simulink library "LibFactorGraph"  (Simulink 8.3)
settings: Solver=ode45  StartTime=0.0  StopTime=10.0  RelTol=1e-3
undefined symbols (not defined in the file or in its folder): bV, epsVal, eu, fcn, fP_0, fV, Hin_0, L_0, Nit_0, P_0, xi
libraries: LibFactorGraph x357
(part 3 of 4)

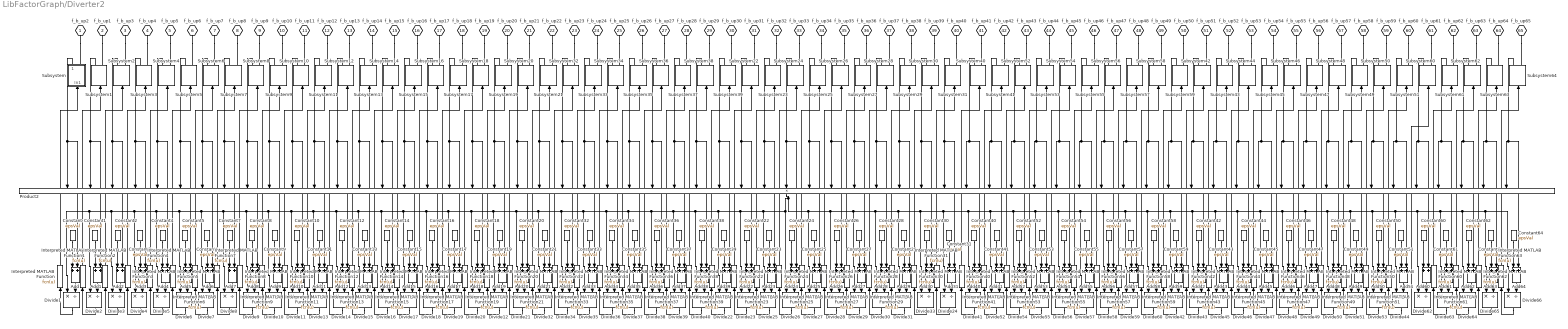
== system LibFactorGraph/Diverter2 ==
  Add{,1..64} (65 alike) : Sum
  Constant{,1..64} (65 alike) : Constant  Value=epsVal
  Divide{1..60,62..66} (65 alike) : Product  Inputs=*/
  Interpreted MATLAB Function{,1..63} (64 alike) : MATLABFcn  MATLABFcn=fcn(u)  Output1D=off
  Product2 : Product  Inputs=65  RndMeth=Zero
  Subsystem : Subsystem
  Subsystem{1..64} (64 alike) : LibFactorGraph/Diverter2/Subsystem
  f_b_up2 : PMIOPort  Port=1  Side=Left
  f_b_up1 : PMIOPort  Port=2  Side=Right
  f_b_up3 : PMIOPort  Port=3  Side=Left
  f_b_up4 : PMIOPort  Port=4  Side=Right
  f_b_up5 : PMIOPort  Port=5  Side=Left
  f_b_up6 : PMIOPort  Port=6  Side=Right
  f_b_up7 : PMIOPort  Port=7  Side=Left
  f_b_up8 : PMIOPort  Port=8  Side=Right
  f_b_up9 : PMIOPort  Port=9  Side=Left
  f_b_up10 : PMIOPort  Port=10  Side=Right
  f_b_up11 : PMIOPort  Port=11  Side=Left
  f_b_up12 : PMIOPort  Port=12  Side=Right
  f_b_up13 : PMIOPort  Port=13  Side=Left
  f_b_up14 : PMIOPort  Port=14  Side=Right
  f_b_up15 : PMIOPort  Port=15  Side=Left
  f_b_up16 : PMIOPort  Port=16  Side=Right
  f_b_up17 : PMIOPort  Port=17  Side=Left
  f_b_up18 : PMIOPort  Port=18  Side=Right
  f_b_up19 : PMIOPort  Port=19  Side=Left
  f_b_up20 : PMIOPort  Port=20  Side=Right
  f_b_up21 : PMIOPort  Port=21  Side=Left
  f_b_up22 : PMIOPort  Port=22  Side=Right
  f_b_up23 : PMIOPort  Port=23  Side=Left
  f_b_up24 : PMIOPort  Port=24  Side=Right
  f_b_up25 : PMIOPort  Port=25  Side=Left
  f_b_up26 : PMIOPort  Port=26  Side=Right
  f_b_up27 : PMIOPort  Port=27  Side=Left
  f_b_up28 : PMIOPort  Port=28  Side=Right
  f_b_up29 : PMIOPort  Port=29  Side=Left
  f_b_up30 : PMIOPort  Port=30  Side=Right
  f_b_up31 : PMIOPort  Port=31  Side=Left
  f_b_up32 : PMIOPort  Port=32  Side=Right
  f_b_up33 : PMIOPort  Port=33  Side=Left
  f_b_up34 : PMIOPort  Port=34  Side=Right
  f_b_up35 : PMIOPort  Port=35  Side=Left
  f_b_up36 : PMIOPort  Port=36  Side=Right
  f_b_up37 : PMIOPort  Port=37  Side=Left
  f_b_up38 : PMIOPort  Port=38  Side=Right
  f_b_up39 : PMIOPort  Port=39  Side=Left
  f_b_up40 : PMIOPort  Port=40  Side=Right
  f_b_up41 : PMIOPort  Port=41  Side=Left
  f_b_up42 : PMIOPort  Port=42  Side=Right
  f_b_up43 : PMIOPort  Port=43  Side=Left
  f_b_up44 : PMIOPort  Port=44  Side=Right
  f_b_up45 : PMIOPort  Port=45  Side=Left
  f_b_up46 : PMIOPort  Port=46  Side=Right
  f_b_up47 : PMIOPort  Port=47  Side=Left
  f_b_up48 : PMIOPort  Port=48  Side=Right
  f_b_up49 : PMIOPort  Port=49  Side=Left
  f_b_up50 : PMIOPort  Port=50  Side=Right
  f_b_up51 : PMIOPort  Port=51  Side=Left
  f_b_up52 : PMIOPort  Port=52  Side=Right
  f_b_up53 : PMIOPort  Port=53  Side=Left
  f_b_up54 : PMIOPort  Port=54  Side=Right
  f_b_up55 : PMIOPort  Port=55  Side=Left
  f_b_up56 : PMIOPort  Port=56  Side=Right
  f_b_up57 : PMIOPort  Port=57  Side=Left
  f_b_up58 : PMIOPort  Port=58  Side=Right
  f_b_up59 : PMIOPort  Port=59  Side=Left
  f_b_up60 : PMIOPort  Port=60  Side=Right
  f_b_up61 : PMIOPort  Port=61  Side=Left
  f_b_up62 : PMIOPort  Port=62  Side=Right
  f_b_up63 : PMIOPort  Port=63  Side=Left
  f_b_up64 : PMIOPort  Port=64  Side=Right
  f_b_up65 : PMIOPort  Port=65  Side=Left
  wires:
  Divide1/1 -> Interpreted MATLAB Function/1
  Subsystem/1(Out1) -> Product2/1, Add/2
  Interpreted MATLAB Function/1 -> Subsystem/1(In1)
  Add/1 -> Divide1/2
  Constant/1 -> Add/1
  Divide2/1 -> Interpreted MATLAB Function1/1
  Subsystem1/1 -> Product2/2, Add1/2
  Interpreted MATLAB Function1/1 -> Subsystem1/1
  Add1/1 -> Divide2/2
  Constant1/1 -> Add1/1
  Product2/1 -> Divide25/1, Divide23/1, Divide22/1, Divide40/1, Divide39/1, Divide38/1, Divide37/1, Divide36/1, Divide35/1, Divide34/1, Divide32/1, Divide21/1, Divide12/1, Divide20/1, Divide19/1, Divide18/1, Divide17/1, Divide16/1, Divide15/1, Divide14/1, Divide13/1, Divide11/1, Divide10/1, Divide9/1, Divide8/1, Divide7/1, Divide6/1, Divide5/1, Divide4/1, Divide3/1, Divide2/1, Divide1/1, Divide26/1, Divide27/1, Divide28/1, Divide29/1, Divide30/1, Divide31/1, Divide33/1, Divide24/1, Divide41/1, Divide52/1, Divide54/1, Divide55/1, Divide56/1, Divide58/1, Divide59/1, Divide60/1, Divide42/1, Divide43/1, Divide45/1, Divide46/1, Divide47/1, Divide48/1, Divide49/1, Divide50/1, Divide51/1, Divide53/1, Divide44/1, Divide62/1, Divide63/1, Divide64/1, Divide65/1, Divide66/1, Divide57/1
  Divide3/1 -> Interpreted MATLAB Function2/1
  Subsystem2/1 -> Product2/3, Add2/2
  Interpreted MATLAB Function2/1 -> Subsystem2/1
  Add2/1 -> Divide3/2
  Constant2/1 -> Add2/1
  Divide4/1 -> Interpreted MATLAB Function3/1
  Subsystem3/1 -> Product2/4, Add3/2
  Interpreted MATLAB Function3/1 -> Subsystem3/1
  Add3/1 -> Divide4/2
  Constant3/1 -> Add3/1
  Divide5/1 -> Interpreted MATLAB Function4/1
  Subsystem4/1 -> Product2/5, Add4/2
  Interpreted MATLAB Function4/1 -> Subsystem4/1
  Add4/1 -> Divide5/2
  Constant4/1 -> Add4/1
  Divide6/1 -> Interpreted MATLAB Function5/1
  Subsystem5/1 -> Product2/6, Add5/2
  Interpreted MATLAB Function5/1 -> Subsystem5/1
  Add5/1 -> Divide6/2
  Constant5/1 -> Add5/1
  Divide7/1 -> Interpreted MATLAB Function6/1
  Subsystem6/1 -> Product2/7, Add6/2
  Interpreted MATLAB Function6/1 -> Subsystem6/1
  Add6/1 -> Divide7/2
  Constant6/1 -> Add6/1
  Divide8/1 -> Interpreted MATLAB Function7/1
  Subsystem7/1 -> Product2/8, Add7/2
  Interpreted MATLAB Function7/1 -> Subsystem7/1
  Add7/1 -> Divide8/2
  Constant7/1 -> Add7/1
  Divide9/1 -> Interpreted MATLAB Function8/1
  Subsystem8/1 -> Product2/9, Add8/2
  Interpreted MATLAB Function8/1 -> Subsystem8/1
  Add8/1 -> Divide9/2
  Constant8/1 -> Add8/1
  Divide10/1 -> Interpreted MATLAB Function9/1
  Subsystem9/1 -> Product2/10, Add9/2
  Interpreted MATLAB Function9/1 -> Subsystem9/1
  Add9/1 -> Divide10/2
  Constant9/1 -> Add9/1
  Divide11/1 -> Interpreted MATLAB Function10/1
  Subsystem10/1 -> Product2/11, Add10/2
  Interpreted MATLAB Function10/1 -> Subsystem10/1
  Add10/1 -> Divide11/2
  Constant10/1 -> Add10/1
  Divide13/1 -> Interpreted MATLAB Function11/1
  Subsystem11/1 -> Product2/12, Add11/2
  Interpreted MATLAB Function11/1 -> Subsystem11/1
  Add11/1 -> Divide13/2
  Constant11/1 -> Add11/1
  Divide14/1 -> Interpreted MATLAB Function12/1
  Subsystem12/1 -> Product2/13, Add12/2
  Interpreted MATLAB Function12/1 -> Subsystem12/1
  Add12/1 -> Divide14/2
  Constant12/1 -> Add12/1
  Divide15/1 -> Interpreted MATLAB Function13/1
  Subsystem13/1 -> Product2/14, Add13/2
  Interpreted MATLAB Function13/1 -> Subsystem13/1
  Add13/1 -> Divide15/2
  Constant13/1 -> Add13/1
  Divide16/1 -> Interpreted MATLAB Function14/1
  Subsystem14/1 -> Product2/15, Add14/2
  Interpreted MATLAB Function14/1 -> Subsystem14/1
  Add14/1 -> Divide16/2
  Constant14/1 -> Add14/1
  Divide17/1 -> Interpreted MATLAB Function15/1
  Subsystem15/1 -> Product2/16, Add15/2
  Interpreted MATLAB Function15/1 -> Subsystem15/1
  Add15/1 -> Divide17/2
  Constant15/1 -> Add15/1
  Divide18/1 -> Interpreted MATLAB Function16/1
  Subsystem16/1 -> Product2/17, Add16/2
  Interpreted MATLAB Function16/1 -> Subsystem16/1
  Add16/1 -> Divide18/2
  Constant16/1 -> Add16/1
  Divide19/1 -> Interpreted MATLAB Function17/1
  Subsystem17/1 -> Product2/18, Add17/2
  Interpreted MATLAB Function17/1 -> Subsystem17/1
  Add17/1 -> Divide19/2
  Constant17/1 -> Add17/1
  Divide20/1 -> Interpreted MATLAB Function18/1
  Subsystem18/1 -> Product2/19, Add18/2
  Interpreted MATLAB Function18/1 -> Subsystem18/1
  Add18/1 -> Divide20/2
  Constant18/1 -> Add18/1
  Divide12/1 -> Interpreted MATLAB Function19/1
  Subsystem19/1 -> Product2/20, Add19/2
  Interpreted MATLAB Function19/1 -> Subsystem19/1
  Add19/1 -> Divide12/2
  Constant19/1 -> Add19/1
  Divide21/1 -> Interpreted MATLAB Function20/1
  Subsystem20/1 -> Product2/21, Add20/2
  Interpreted MATLAB Function20/1 -> Subsystem20/1
  Add20/1 -> Divide21/2
  Constant20/1 -> Add20/1
  Divide32/1 -> Interpreted MATLAB Function21/1
  Subsystem21/1 -> Product2/22, Add21/2
  Interpreted MATLAB Function21/1 -> Subsystem21/1
  Add21/1 -> Divide32/2
  Constant21/1 -> Add21/1
  Divide34/1 -> Interpreted MATLAB Function32/1
  Subsystem32/1 -> Product2/23, Add32/2
  Interpreted MATLAB Function32/1 -> Subsystem32/1
  Add32/1 -> Divide34/2
  Constant32/1 -> Add32/1
  Divide35/1 -> Interpreted MATLAB Function33/1
  Subsystem33/1 -> Product2/24, Add33/2
  Interpreted MATLAB Function33/1 -> Subsystem33/1
  Add33/1 -> Divide35/2
  Constant33/1 -> Add33/1
  Divide36/1 -> Interpreted MATLAB Function34/1
  Subsystem34/1 -> Product2/25, Add34/2
  Interpreted MATLAB Function34/1 -> Subsystem34/1
  Add34/1 -> Divide36/2
  Constant34/1 -> Add34/1
  Divide37/1 -> Interpreted MATLAB Function35/1
  Subsystem35/1 -> Product2/26, Add35/2
  Interpreted MATLAB Function35/1 -> Subsystem35/1
  Add35/1 -> Divide37/2
  Constant35/1 -> Add35/1
  Divide38/1 -> Interpreted MATLAB Function36/1
  Subsystem36/1 -> Product2/27, Add36/2
  Interpreted MATLAB Function36/1 -> Subsystem36/1
  Add36/1 -> Divide38/2
  Constant36/1 -> Add36/1
  Divide39/1 -> Interpreted MATLAB Function37/1
  Subsystem37/1 -> Product2/28, Add37/2
  Interpreted MATLAB Function37/1 -> Subsystem37/1
  Add37/1 -> Divide39/2
  Constant37/1 -> Add37/1
  Divide40/1 -> Interpreted MATLAB Function38/1
  Subsystem38/1 -> Product2/29, Add38/2
  Interpreted MATLAB Function38/1 -> Subsystem38/1
  Add38/1 -> Divide40/2
  Constant38/1 -> Add38/1
  Divide22/1 -> Interpreted MATLAB Function39/1
  Subsystem39/1 -> Product2/30, Add39/2
  Interpreted MATLAB Function39/1 -> Subsystem39/1
  Add39/1 -> Divide22/2
  Constant39/1 -> Add39/1
  Divide23/1 -> Interpreted MATLAB Function22/1
  Subsystem22/1 -> Product2/31, Add22/2
  Interpreted MATLAB Function22/1 -> Subsystem22/1
  Add22/1 -> Divide23/2
  Constant22/1 -> Add22/1
  Divide25/1 -> Interpreted MATLAB Function23/1
  Subsystem23/1 -> Product2/32, Add23/2
  Interpreted MATLAB Function23/1 -> Subsystem23/1
  Add23/1 -> Divide25/2
  Constant23/1 -> Add23/1
  Divide26/1 -> Interpreted MATLAB Function24/1
  Subsystem24/1 -> Product2/33, Add24/2
  Interpreted MATLAB Function24/1 -> Subsystem24/1
  Add24/1 -> Divide26/2
  Constant24/1 -> Add24/1
  Divide27/1 -> Interpreted MATLAB Function25/1
  Subsystem25/1 -> Product2/34, Add25/2
  Interpreted MATLAB Function25/1 -> Subsystem25/1
  Add25/1 -> Divide27/2
  Constant25/1 -> Add25/1
  Divide28/1 -> Interpreted MATLAB Function26/1
  Subsystem26/1 -> Product2/35, Add26/2
  Interpreted MATLAB Function26/1 -> Subsystem26/1
  Add26/1 -> Divide28/2
  Constant26/1 -> Add26/1
  Divide29/1 -> Interpreted MATLAB Function27/1
  Subsystem27/1 -> Product2/36, Add27/2
  Interpreted MATLAB Function27/1 -> Subsystem27/1
  Add27/1 -> Divide29/2
  Constant27/1 -> Add27/1
  Divide30/1 -> Interpreted MATLAB Function28/1
  Subsystem28/1 -> Product2/37, Add28/2
  Interpreted MATLAB Function28/1 -> Subsystem28/1
  Add28/1 -> Divide30/2
  Constant28/1 -> Add28/1
  Divide31/1 -> Interpreted MATLAB Function29/1
  Subsystem29/1 -> Product2/38, Add29/2
  Interpreted MATLAB Function29/1 -> Subsystem29/1
  Add29/1 -> Divide31/2
  Constant29/1 -> Add29/1
  Divide33/1 -> Interpreted MATLAB Function30/1
  Subsystem30/1 -> Product2/39, Add30/2
  Interpreted MATLAB Function30/1 -> Subsystem30/1
  Add30/1 -> Divide33/2
  Constant30/1 -> Add30/1
  Divide24/1 -> Interpreted MATLAB Function31/1
  Subsystem31/1 -> Product2/40, Add31/2
  Interpreted MATLAB Function31/1 -> Subsystem31/1
  Add31/1 -> Divide24/2
  Constant31/1 -> Add31/1
  Divide41/1 -> Interpreted MATLAB Function40/1
  Subsystem40/1 -> Product2/41, Add40/2
  Interpreted MATLAB Function40/1 -> Subsystem40/1
  Add40/1 -> Divide41/2
  Constant40/1 -> Add40/1
  Divide52/1 -> Interpreted MATLAB Function41/1
  Subsystem41/1 -> Product2/42, Add41/2
  Interpreted MATLAB Function41/1 -> Subsystem41/1
  Add41/1 -> Divide52/2
  Constant41/1 -> Add41/1
  Divide54/1 -> Interpreted MATLAB Function52/1
  Subsystem52/1 -> Product2/43, Add52/2
  Interpreted MATLAB Function52/1 -> Subsystem52/1
  Add52/1 -> Divide54/2
  Constant52/1 -> Add52/1
  Divide55/1 -> Interpreted MATLAB Function53/1
  Subsystem53/1 -> Product2/44, Add53/2
  Interpreted MATLAB Function53/1 -> Subsystem53/1
  Add53/1 -> Divide55/2
  Constant53/1 -> Add53/1
  Divide56/1 -> Interpreted MATLAB Function54/1
  Subsystem54/1 -> Product2/45, Add54/2
  Interpreted MATLAB Function54/1 -> Subsystem54/1
  Add54/1 -> Divide56/2
  Constant54/1 -> Add54/1
  Divide57/1 -> Interpreted MATLAB Function55/1
  Subsystem55/1 -> Product2/46, Add55/2
  Interpreted MATLAB Function55/1 -> Subsystem55/1
  Add55/1 -> Divide57/2
  Constant55/1 -> Add55/1
  Divide58/1 -> Interpreted MATLAB Function56/1
  Subsystem56/1 -> Product2/47, Add56/2
  Interpreted MATLAB Function56/1 -> Subsystem56/1
  Add56/1 -> Divide58/2
  Constant56/1 -> Add56/1
  Divide59/1 -> Interpreted MATLAB Function57/1
  Subsystem57/1 -> Product2/48, Add57/2
  Interpreted MATLAB Function57/1 -> Subsystem57/1
  Add57/1 -> Divide59/2
  Constant57/1 -> Add57/1
  Divide60/1 -> Interpreted MATLAB Function58/1
  Subsystem58/1 -> Product2/49, Add58/2
  Interpreted MATLAB Function58/1 -> Subsystem58/1
  Add58/1 -> Divide60/2
  Constant58/1 -> Add58/1
  Divide42/1 -> Interpreted MATLAB Function59/1
  Subsystem59/1 -> Product2/50, Add59/2
  Interpreted MATLAB Function59/1 -> Subsystem59/1
  Add59/1 -> Divide42/2
  Constant59/1 -> Add59/1
  Divide43/1 -> Interpreted MATLAB Function42/1
  Subsystem42/1 -> Product2/51, Add42/2
  Interpreted MATLAB Function42/1 -> Subsystem42/1
  Add42/1 -> Divide43/2
  Constant42/1 -> Add42/1
  Divide45/1 -> Interpreted MATLAB Function43/1
  Subsystem43/1 -> Product2/52, Add43/2
  Interpreted MATLAB Function43/1 -> Subsystem43/1
  Add43/1 -> Divide45/2
  Constant43/1 -> Add43/1
  Divide46/1 -> Interpreted MATLAB Function44/1
  Subsystem44/1 -> Product2/53, Add44/2
  Interpreted MATLAB Function44/1 -> Subsystem44/1
  Add44/1 -> Divide46/2
  Constant44/1 -> Add44/1
  Divide47/1 -> Interpreted MATLAB Function45/1
  Subsystem45/1 -> Product2/54, Add45/2
  Interpreted MATLAB Function45/1 -> Subsystem45/1
  Add45/1 -> Divide47/2
  Constant45/1 -> Add45/1
  Divide48/1 -> Interpreted MATLAB Function46/1
  Subsystem46/1 -> Product2/55, Add46/2
  Interpreted MATLAB Function46/1 -> Subsystem46/1
  Add46/1 -> Divide48/2
  Constant46/1 -> Add46/1
  Divide49/1 -> Interpreted MATLAB Function47/1
  Subsystem47/1 -> Product2/56, Add47/2
  Interpreted MATLAB Function47/1 -> Subsystem47/1
  Add47/1 -> Divide49/2
  Constant47/1 -> Add47/1
  Divide50/1 -> Interpreted MATLAB Function48/1
  Subsystem48/1 -> Product2/57, Add48/2
  Interpreted MATLAB Function48/1 -> Subsystem48/1
  Add48/1 -> Divide50/2
  Constant48/1 -> Add48/1
  Divide51/1 -> Interpreted MATLAB Function49/1
  Subsystem49/1 -> Product2/58, Add49/2
  Interpreted MATLAB Function49/1 -> Subsystem49/1
  Add49/1 -> Divide51/2
  Constant49/1 -> Add49/1
  Divide53/1 -> Interpreted MATLAB Function50/1
  Subsystem50/1 -> Product2/59, Add50/2
  Interpreted MATLAB Function50/1 -> Subsystem50/1
  Add50/1 -> Divide53/2
  Constant50/1 -> Add50/1
  Divide44/1 -> Interpreted MATLAB Function51/1
  Subsystem51/1 -> Product2/60, Add51/2
  Interpreted MATLAB Function51/1 -> Subsystem51/1
  Add51/1 -> Divide44/2
  Constant51/1 -> Add51/1
  Subsystem60/1 -> Product2/61, Add60/2
  Divide62/1 -> Subsystem60/1
  Add60/1 -> Divide62/2
  Constant60/1 -> Add60/1
  Divide63/1 -> Interpreted MATLAB Function60/1
  Subsystem61/1 -> Product2/62, Add61/2
  Interpreted MATLAB Function60/1 -> Subsystem61/1
  Add61/1 -> Divide63/2
  Constant61/1 -> Add61/1
  Divide64/1 -> Interpreted MATLAB Function61/1
  Subsystem62/1 -> Product2/63, Add62/2
  Interpreted MATLAB Function61/1 -> Subsystem62/1
  Add62/1 -> Divide64/2
  Constant62/1 -> Add62/1
  Divide65/1 -> Interpreted MATLAB Function62/1
  Subsystem63/1 -> Product2/64, Add63/2
  Interpreted MATLAB Function62/1 -> Subsystem63/1
  Add63/1 -> Divide65/2
  Constant63/1 -> Add63/1
  Divide66/1 -> Interpreted MATLAB Function63/1
  Subsystem64/1 -> Product2/65, Add64/2
  Interpreted MATLAB Function63/1 -> Subsystem64/1
  Add64/1 -> Divide66/2
  Constant64/1 -> Add64/1
  connections:
  f_b_up2/RConn1 -- Subsystem/RConn1
  f_b_up1/RConn1 -- Subsystem1/RConn1
  f_b_up3/RConn1 -- Subsystem2/RConn1
  f_b_up4/RConn1 -- Subsystem3/RConn1
  f_b_up5/RConn1 -- Subsystem4/RConn1
  f_b_up7/RConn1 -- Subsystem6/RConn1
  f_b_up6/RConn1 -- Subsystem5/RConn1
  f_b_up10/RConn1 -- Subsystem9/RConn1
  f_b_up8/RConn1 -- Subsystem7/RConn1
  f_b_up9/RConn1 -- Subsystem8/RConn1
  f_b_up16/RConn1 -- Subsystem15/RConn1
  f_b_up14/RConn1 -- Subsystem13/RConn1
  f_b_up12/RConn1 -- Subsystem11/RConn1
  f_b_up15/RConn1 -- Subsystem14/RConn1
  f_b_up19/RConn1 -- Subsystem18/RConn1
  f_b_up18/RConn1 -- Subsystem17/RConn1
  f_b_up11/RConn1 -- Subsystem10/RConn1
  f_b_up17/RConn1 -- Subsystem16/RConn1
  f_b_up20/RConn1 -- Subsystem19/RConn1
  f_b_up13/RConn1 -- Subsystem12/RConn1
  f_b_up36/RConn1 -- Subsystem27/RConn1
  f_b_up38/RConn1 -- Subsystem29/RConn1
  f_b_up26/RConn1 -- Subsystem35/RConn1
  f_b_up39/RConn1 -- Subsystem30/RConn1
  f_b_up23/RConn1 -- Subsystem32/RConn1
  f_b_up34/RConn1 -- Subsystem25/RConn1
  f_b_up27/RConn1 -- Subsystem36/RConn1
  f_b_up25/RConn1 -- Subsystem34/RConn1
  f_b_up31/RConn1 -- Subsystem22/RConn1
  f_b_up24/RConn1 -- Subsystem33/RConn1
  f_b_up22/RConn1 -- Subsystem21/RConn1
  f_b_up28/RConn1 -- Subsystem37/RConn1
  f_b_up37/RConn1 -- Subsystem28/RConn1
  f_b_up33/RConn1 -- Subsystem24/RConn1
  f_b_up30/RConn1 -- Subsystem39/RConn1
  f_b_up35/RConn1 -- Subsystem26/RConn1
  f_b_up21/RConn1 -- Subsystem20/RConn1
  f_b_up32/RConn1 -- Subsystem23/RConn1
  f_b_up40/RConn1 -- Subsystem31/RConn1
  f_b_up29/RConn1 -- Subsystem38/RConn1
  f_b_up56/RConn1 -- Subsystem47/RConn1
  f_b_up58/RConn1 -- Subsystem49/RConn1
  f_b_up46/RConn1 -- Subsystem55/RConn1
  f_b_up59/RConn1 -- Subsystem50/RConn1
  f_b_up43/RConn1 -- Subsystem52/RConn1
  f_b_up54/RConn1 -- Subsystem45/RConn1
  f_b_up47/RConn1 -- Subsystem56/RConn1
  f_b_up45/RConn1 -- Subsystem54/RConn1
  f_b_up51/RConn1 -- Subsystem42/RConn1
  f_b_up44/RConn1 -- Subsystem53/RConn1
  f_b_up42/RConn1 -- Subsystem41/RConn1
  f_b_up48/RConn1 -- Subsystem57/RConn1
  f_b_up57/RConn1 -- Subsystem48/RConn1
  f_b_up53/RConn1 -- Subsystem44/RConn1
  f_b_up50/RConn1 -- Subsystem59/RConn1
  f_b_up55/RConn1 -- Subsystem46/RConn1
  f_b_up41/RConn1 -- Subsystem40/RConn1
  f_b_up52/RConn1 -- Subsystem43/RConn1
  f_b_up60/RConn1 -- Subsystem51/RConn1
  f_b_up49/RConn1 -- Subsystem58/RConn1
  f_b_up63/RConn1 -- Subsystem62/RConn1
  f_b_up64/RConn1 -- Subsystem63/RConn1
  f_b_up62/RConn1 -- Subsystem61/RConn1
  f_b_up65/RConn1 -- Subsystem64/RConn1
  f_b_up61/RConn1 -- Subsystem60/RConn1

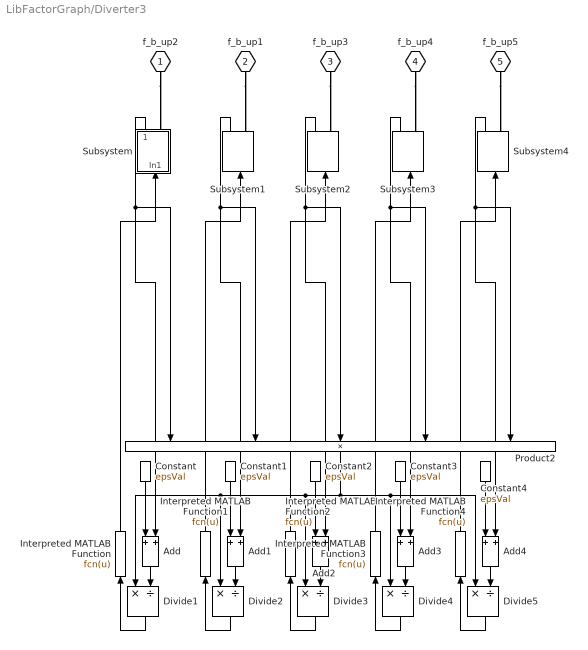
== system LibFactorGraph/Diverter3 ==
  Add{,1..4} (5 alike) : Sum
  Constant{,1..4} (5 alike) : Constant  Value=epsVal
  Divide{1..5} (5 alike) : Product  Inputs=*/
  Interpreted MATLAB Function{,1..4} (5 alike) : MATLABFcn  MATLABFcn=fcn(u)  Output1D=off
  Product2 : Product  Inputs=5  RndMeth=Zero
  Subsystem : Subsystem
  Subsystem{1..4} (4 alike) : LibFactorGraph/Diverter3/Subsystem
  f_b_up2 : PMIOPort  Port=1  Side=Left
  f_b_up1 : PMIOPort  Port=2  Side=Right
  f_b_up3 : PMIOPort  Port=3  Side=Left
  f_b_up4 : PMIOPort  Port=4  Side=Right
  f_b_up5 : PMIOPort  Port=5  Side=Left
  wires:
  Constant/1 -> Add/1
  Add/1 -> Divide1/2
  Interpreted MATLAB Function/1 -> Subsystem/1(In1)
  Subsystem/1(Out1) -> Add/2, Product2/1
  Divide1/1 -> Interpreted MATLAB Function/1
  Constant1/1 -> Add1/1
  Add1/1 -> Divide2/2
  Interpreted MATLAB Function1/1 -> Subsystem1/1
  Subsystem1/1 -> Product2/2, Add1/2
  Divide2/1 -> Interpreted MATLAB Function1/1
  Constant2/1 -> Add2/1
  Add2/1 -> Divide3/2
  Interpreted MATLAB Function2/1 -> Subsystem2/1
  Subsystem2/1 -> Product2/3, Add2/2
  Divide3/1 -> Interpreted MATLAB Function2/1
  Constant3/1 -> Add3/1
  Add3/1 -> Divide4/2
  Interpreted MATLAB Function3/1 -> Subsystem3/1
  Subsystem3/1 -> Product2/4, Add3/2
  Divide4/1 -> Interpreted MATLAB Function3/1
  Product2/1 -> Divide2/1, Divide1/1, Divide3/1, Divide5/1, Divide4/1
  Constant4/1 -> Add4/1
  Add4/1 -> Divide5/2
  Interpreted MATLAB Function4/1 -> Subsystem4/1
  Subsystem4/1 -> Product2/5, Add4/2
  Divide5/1 -> Interpreted MATLAB Function4/1
  connections:
  f_b_up2/RConn1 -- Subsystem/RConn1
  f_b_up1/RConn1 -- Subsystem1/RConn1
  f_b_up3/RConn1 -- Subsystem2/RConn1
  f_b_up4/RConn1 -- Subsystem3/RConn1
  f_b_up5/RConn1 -- Subsystem4/RConn1

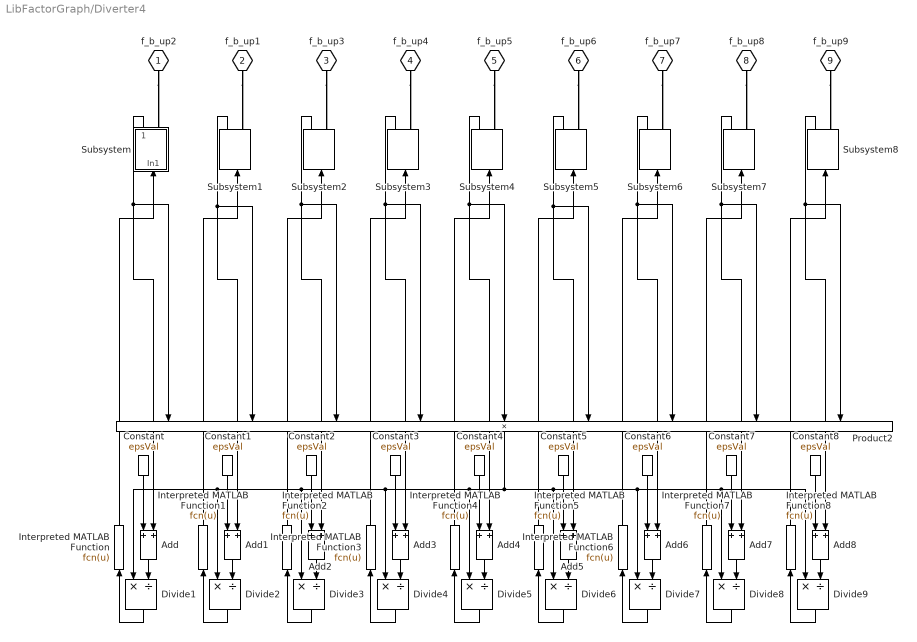
== system LibFactorGraph/Diverter4 ==
  Add{,1..8} (9 alike) : Sum
  Constant{,1..8} (9 alike) : Constant  Value=epsVal
  Divide{1..9} (9 alike) : Product  Inputs=*/
  Interpreted MATLAB Function{,1..8} (9 alike) : MATLABFcn  MATLABFcn=fcn(u)  Output1D=off
  Product2 : Product  Inputs=9  RndMeth=Zero
  Subsystem : Subsystem
  Subsystem{1..3,5..8} (7 alike) : LibFactorGraph/Diverter3/Subsystem
  Subsystem4 : LibFactorGraph/Diverter4/Subsystem
  f_b_up2 : PMIOPort  Port=1  Side=Left
  f_b_up1 : PMIOPort  Port=2  Side=Right
  f_b_up3 : PMIOPort  Port=3  Side=Left
  f_b_up4 : PMIOPort  Port=4  Side=Right
  f_b_up5 : PMIOPort  Port=5  Side=Left
  f_b_up6 : PMIOPort  Port=6  Side=Right
  f_b_up7 : PMIOPort  Port=7  Side=Left
  f_b_up8 : PMIOPort  Port=8  Side=Right
  f_b_up9 : PMIOPort  Port=9  Side=Left
  wires:
  Divide4/1 -> Interpreted MATLAB Function3/1
  Subsystem3/1 -> Add3/2, Product2/4
  Interpreted MATLAB Function3/1 -> Subsystem3/1
  Add3/1 -> Divide4/2
  Constant3/1 -> Add3/1
  Divide3/1 -> Interpreted MATLAB Function2/1
  Subsystem2/1 -> Add2/2, Product2/3
  Interpreted MATLAB Function2/1 -> Subsystem2/1
  Add2/1 -> Divide3/2
  Constant2/1 -> Add2/1
  Divide2/1 -> Interpreted MATLAB Function1/1
  Subsystem1/1 -> Product2/2, Add1/2
  Interpreted MATLAB Function1/1 -> Subsystem1/1
  Add1/1 -> Divide2/2
  Constant1/1 -> Add1/1
  Divide1/1 -> Interpreted MATLAB Function/1
  Subsystem/1(Out1) -> Product2/1, Add/2
  Interpreted MATLAB Function/1 -> Subsystem/1(In1)
  Add/1 -> Divide1/2
  Constant/1 -> Add/1
  Divide8/1 -> Interpreted MATLAB Function7/1
  Subsystem7/1 -> Product2/8, Add7/2
  Interpreted MATLAB Function7/1 -> Subsystem7/1
  Add7/1 -> Divide8/2
  Constant7/1 -> Add7/1
  Divide7/1 -> Interpreted MATLAB Function6/1
  Subsystem6/1 -> Product2/7, Add6/2
  Interpreted MATLAB Function6/1 -> Subsystem6/1
  Add6/1 -> Divide7/2
  Constant6/1 -> Add6/1
  Divide6/1 -> Interpreted MATLAB Function5/1
  Subsystem5/1 -> Product2/6, Add5/2
  Interpreted MATLAB Function5/1 -> Subsystem5/1
  Add5/1 -> Divide6/2
  Constant5/1 -> Add5/1
  Divide5/1 -> Interpreted MATLAB Function4/1
  Subsystem4/1 -> Product2/5, Add4/2
  Interpreted MATLAB Function4/1 -> Subsystem4/1
  Add4/1 -> Divide5/2
  Constant4/1 -> Add4/1
  Divide9/1 -> Interpreted MATLAB Function8/1
  Subsystem8/1 -> Product2/9, Add8/2
  Interpreted MATLAB Function8/1 -> Subsystem8/1
  Add8/1 -> Divide9/2
  Constant8/1 -> Add8/1
  Product2/1 -> Divide5/1, Divide1/1, Divide2/1, Divide3/1, Divide4/1, Divide9/1, Divide8/1, Divide7/1, Divide6/1
  connections:
  f_b_up4/RConn1 -- Subsystem3/RConn1
  f_b_up3/RConn1 -- Subsystem2/RConn1
  f_b_up1/RConn1 -- Subsystem1/RConn1
  f_b_up2/RConn1 -- Subsystem/RConn1
  f_b_up5/RConn1 -- Subsystem4/RConn1
  f_b_up6/RConn1 -- Subsystem5/RConn1
  f_b_up8/RConn1 -- Subsystem7/RConn1
  f_b_up7/RConn1 -- Subsystem6/RConn1
  f_b_up9/RConn1 -- Subsystem8/RConn1

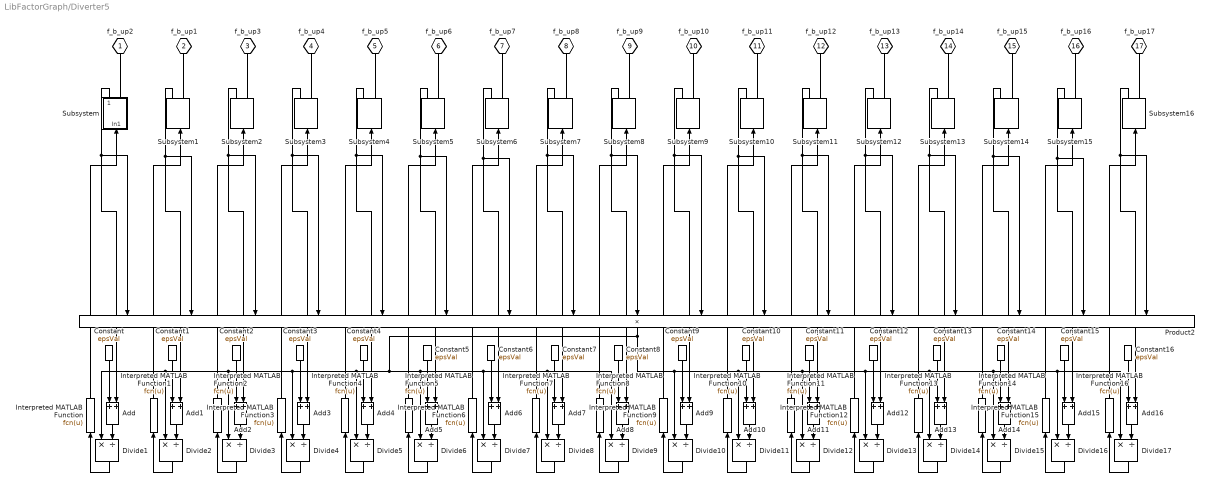
== system LibFactorGraph/Diverter5 ==
  Add{,1..16} (17 alike) : Sum
  Constant{,1..16} (17 alike) : Constant  Value=epsVal
  Divide{1..17} (17 alike) : Product  Inputs=*/
  Interpreted MATLAB Function{,1..16} (17 alike) : MATLABFcn  MATLABFcn=fcn(u)  Output1D=off
  Product2 : Product  Inputs=17  RndMeth=Zero
  Subsystem : Subsystem
  Subsystem{1..3,5..8,10..12,14..16} (13 alike) : LibFactorGraph/Diverter3/Subsystem
  Subsystem13 : LibFactorGraph/Diverter4/Subsystem
  Subsystem4 : LibFactorGraph/Diverter4/Subsystem
  Subsystem9 : LibFactorGraph/Diverter5/Subsystem
  f_b_up2 : PMIOPort  Port=1  Side=Left
  f_b_up1 : PMIOPort  Port=2  Side=Right
  f_b_up3 : PMIOPort  Port=3  Side=Left
  f_b_up4 : PMIOPort  Port=4  Side=Right
  f_b_up5 : PMIOPort  Port=5  Side=Left
  f_b_up6 : PMIOPort  Port=6  Side=Right
  f_b_up7 : PMIOPort  Port=7  Side=Left
  f_b_up8 : PMIOPort  Port=8  Side=Right
  f_b_up9 : PMIOPort  Port=9  Side=Left
  f_b_up10 : PMIOPort  Port=10  Side=Right
  f_b_up11 : PMIOPort  Port=11  Side=Left
  f_b_up12 : PMIOPort  Port=12  Side=Right
  f_b_up13 : PMIOPort  Port=13  Side=Left
  f_b_up14 : PMIOPort  Port=14  Side=Right
  f_b_up15 : PMIOPort  Port=15  Side=Left
  f_b_up16 : PMIOPort  Port=16  Side=Right
  f_b_up17 : PMIOPort  Port=17  Side=Left
  wires:
  Divide4/1 -> Interpreted MATLAB Function3/1
  Subsystem3/1 -> Add3/2, Product2/4
  Interpreted MATLAB Function3/1 -> Subsystem3/1
  Add3/1 -> Divide4/2
  Constant3/1 -> Add3/1
  Divide3/1 -> Interpreted MATLAB Function2/1
  Subsystem2/1 -> Add2/2, Product2/3
  Interpreted MATLAB Function2/1 -> Subsystem2/1
  Add2/1 -> Divide3/2
  Constant2/1 -> Add2/1
  Divide2/1 -> Interpreted MATLAB Function1/1
  Subsystem1/1 -> Product2/2, Add1/2
  Interpreted MATLAB Function1/1 -> Subsystem1/1
  Add1/1 -> Divide2/2
  Constant1/1 -> Add1/1
  Divide1/1 -> Interpreted MATLAB Function/1
  Subsystem/1(Out1) -> Product2/1, Add/2
  Interpreted MATLAB Function/1 -> Subsystem/1(In1)
  Add/1 -> Divide1/2
  Constant/1 -> Add/1
  Divide8/1 -> Interpreted MATLAB Function7/1
  Subsystem7/1 -> Product2/8, Add7/2
  Interpreted MATLAB Function7/1 -> Subsystem7/1
  Add7/1 -> Divide8/2
  Constant7/1 -> Add7/1
  Divide7/1 -> Interpreted MATLAB Function6/1
  Subsystem6/1 -> Product2/7, Add6/2
  Interpreted MATLAB Function6/1 -> Subsystem6/1
  Add6/1 -> Divide7/2
  Constant6/1 -> Add6/1
  Divide6/1 -> Interpreted MATLAB Function5/1
  Subsystem5/1 -> Product2/6, Add5/2
  Interpreted MATLAB Function5/1 -> Subsystem5/1
  Add5/1 -> Divide6/2
  Constant5/1 -> Add5/1
  Divide5/1 -> Interpreted MATLAB Function4/1
  Subsystem4/1 -> Product2/5, Add4/2
  Interpreted MATLAB Function4/1 -> Subsystem4/1
  Add4/1 -> Divide5/2
  Constant4/1 -> Add4/1
  Divide9/1 -> Interpreted MATLAB Function8/1
  Subsystem8/1 -> Product2/9, Add8/2
  Interpreted MATLAB Function8/1 -> Subsystem8/1
  Add8/1 -> Divide9/2
  Constant8/1 -> Add8/1
  Divide13/1 -> Interpreted MATLAB Function12/1
  Subsystem12/1 -> Product2/13, Add12/2
  Interpreted MATLAB Function12/1 -> Subsystem12/1
  Add12/1 -> Divide13/2
  Constant12/1 -> Add12/1
  Divide12/1 -> Interpreted MATLAB Function11/1
  Subsystem11/1 -> Product2/12, Add11/2
  Interpreted MATLAB Function11/1 -> Subsystem11/1
  Add11/1 -> Divide12/2
  Constant11/1 -> Add11/1
  Divide11/1 -> Interpreted MATLAB Function10/1
  Subsystem10/1 -> Product2/11, Add10/2
  Interpreted MATLAB Function10/1 -> Subsystem10/1
  Add10/1 -> Divide11/2
  Constant10/1 -> Add10/1
  Divide10/1 -> Interpreted MATLAB Function9/1
  Subsystem9/1 -> Product2/10, Add9/2
  Interpreted MATLAB Function9/1 -> Subsystem9/1
  Add9/1 -> Divide10/2
  Constant9/1 -> Add9/1
  Divide17/1 -> Interpreted MATLAB Function16/1
  Subsystem16/1 -> Product2/17, Add16/2
  Interpreted MATLAB Function16/1 -> Subsystem16/1
  Add16/1 -> Divide17/2
  Constant16/1 -> Add16/1
  Divide16/1 -> Interpreted MATLAB Function15/1
  Subsystem15/1 -> Product2/16, Add15/2
  Interpreted MATLAB Function15/1 -> Subsystem15/1
  Add15/1 -> Divide16/2
  Constant15/1 -> Add15/1
  Divide15/1 -> Interpreted MATLAB Function14/1
  Subsystem14/1 -> Product2/15, Add14/2
  Interpreted MATLAB Function14/1 -> Subsystem14/1
  Add14/1 -> Divide15/2
  Constant14/1 -> Add14/1
  Divide14/1 -> Interpreted MATLAB Function13/1
  Subsystem13/1 -> Product2/14, Add13/2
  Interpreted MATLAB Function13/1 -> Subsystem13/1
  Add13/1 -> Divide14/2
  Constant13/1 -> Add13/1
  Product2/1 -> Divide17/1, Divide16/1, Divide15/1, Divide14/1, Divide13/1, Divide12/1, Divide11/1, Divide10/1, Divide5/1, Divide1/1, Divide2/1, Divide3/1, Divide4/1, Divide9/1, Divide8/1, Divide7/1, Divide6/1
  connections:
  f_b_up4/RConn1 -- Subsystem3/RConn1
  f_b_up3/RConn1 -- Subsystem2/RConn1
  f_b_up1/RConn1 -- Subsystem1/RConn1
  f_b_up2/RConn1 -- Subsystem/RConn1
  f_b_up5/RConn1 -- Subsystem4/RConn1
  f_b_up6/RConn1 -- Subsystem5/RConn1
  f_b_up8/RConn1 -- Subsystem7/RConn1
  f_b_up7/RConn1 -- Subsystem6/RConn1
  f_b_up9/RConn1 -- Subsystem8/RConn1
  f_b_up10/RConn1 -- Subsystem9/RConn1
  f_b_up11/RConn1 -- Subsystem10/RConn1
  f_b_up14/RConn1 -- Subsystem13/RConn1
  f_b_up17/RConn1 -- Subsystem16/RConn1
  f_b_up12/RConn1 -- Subsystem11/RConn1
  f_b_up16/RConn1 -- Subsystem15/RConn1
  f_b_up15/RConn1 -- Subsystem14/RConn1
  f_b_up13/RConn1 -- Subsystem12/RConn1

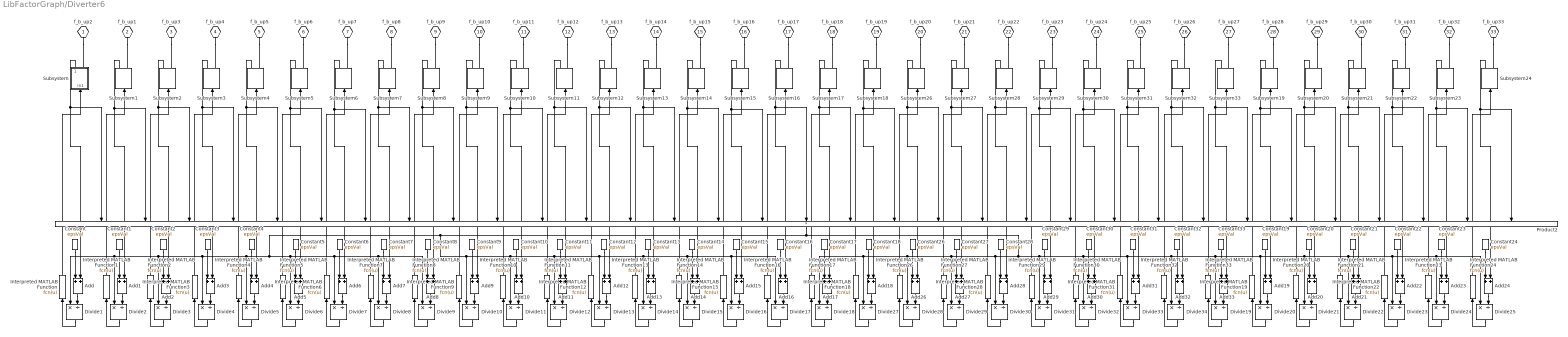
== system LibFactorGraph/Diverter6 ==
  Add{,1..24,26..33} (33 alike) : Sum
  Constant{,1..24,26..33} (33 alike) : Constant  Value=epsVal
  Divide{1..25,27..34} (33 alike) : Product  Inputs=*/
  Interpreted MATLAB Function{,1..24,26..33} (33 alike) : MATLABFcn  MATLABFcn=fcn(u)  Output1D=off
  Product2 : Product  Inputs=33  RndMeth=Zero
  Subsystem : Subsystem
  Subsystem{1..3,5..8,10..12,14..16,18..21,23..24,26..27,29..32} (25 alike) : LibFactorGraph/Diverter3/Subsystem
  Subsystem{4,13,22,28} (4 alike) : LibFactorGraph/Diverter4/Subsystem
  Subsystem17 : LibFactorGraph/Diverter6/Subsystem
  Subsystem33 : LibFactorGraph/Diverter5/Subsystem
  Subsystem9 : LibFactorGraph/Diverter5/Subsystem
  f_b_up2 : PMIOPort  Port=1  Side=Left
  f_b_up1 : PMIOPort  Port=2  Side=Right
  f_b_up3 : PMIOPort  Port=3  Side=Left
  f_b_up4 : PMIOPort  Port=4  Side=Right
  f_b_up5 : PMIOPort  Port=5  Side=Left
  f_b_up6 : PMIOPort  Port=6  Side=Right
  f_b_up7 : PMIOPort  Port=7  Side=Left
  f_b_up8 : PMIOPort  Port=8  Side=Right
  f_b_up9 : PMIOPort  Port=9  Side=Left
  f_b_up10 : PMIOPort  Port=10  Side=Right
  f_b_up11 : PMIOPort  Port=11  Side=Left
  f_b_up12 : PMIOPort  Port=12  Side=Right
  f_b_up13 : PMIOPort  Port=13  Side=Left
  f_b_up14 : PMIOPort  Port=14  Side=Right
  f_b_up15 : PMIOPort  Port=15  Side=Left
  f_b_up16 : PMIOPort  Port=16  Side=Right
  f_b_up17 : PMIOPort  Port=17  Side=Left
  f_b_up18 : PMIOPort  Port=18  Side=Right
  f_b_up19 : PMIOPort  Port=19  Side=Left
  f_b_up20 : PMIOPort  Port=20  Side=Right
  f_b_up21 : PMIOPort  Port=21  Side=Left
  f_b_up22 : PMIOPort  Port=22  Side=Right
  f_b_up23 : PMIOPort  Port=23  Side=Left
  f_b_up24 : PMIOPort  Port=24  Side=Right
  f_b_up25 : PMIOPort  Port=25  Side=Left
  f_b_up26 : PMIOPort  Port=26  Side=Right
  f_b_up27 : PMIOPort  Port=27  Side=Left
  f_b_up28 : PMIOPort  Port=28  Side=Right
  f_b_up29 : PMIOPort  Port=29  Side=Left
  f_b_up30 : PMIOPort  Port=30  Side=Right
  f_b_up31 : PMIOPort  Port=31  Side=Left
  f_b_up32 : PMIOPort  Port=32  Side=Right
  f_b_up33 : PMIOPort  Port=33  Side=Left
  wires:
  Constant13/1 -> Add13/1
  Add13/1 -> Divide14/2
  Interpreted MATLAB Function13/1 -> Subsystem13/1
  Subsystem13/1 -> Add13/2, Product2/14
  Divide14/1 -> Interpreted MATLAB Function13/1
  Constant14/1 -> Add14/1
  Add14/1 -> Divide15/2
  Interpreted MATLAB Function14/1 -> Subsystem14/1
  Subsystem14/1 -> Add14/2, Product2/15
  Divide15/1 -> Interpreted MATLAB Function14/1
  Constant15/1 -> Add15/1
  Add15/1 -> Divide16/2
  Interpreted MATLAB Function15/1 -> Subsystem15/1
  Subsystem15/1 -> Add15/2, Product2/16
  Divide16/1 -> Interpreted MATLAB Function15/1
  Constant16/1 -> Add16/1
  Add16/1 -> Divide17/2
  Interpreted MATLAB Function16/1 -> Subsystem16/1
  Subsystem16/1 -> Add16/2, Product2/17
  Divide17/1 -> Interpreted MATLAB Function16/1
  Constant9/1 -> Add9/1
  Add9/1 -> Divide10/2
  Interpreted MATLAB Function9/1 -> Subsystem9/1
  Subsystem9/1 -> Add9/2, Product2/10
  Divide10/1 -> Interpreted MATLAB Function9/1
  Constant10/1 -> Add10/1
  Add10/1 -> Divide11/2
  Interpreted MATLAB Function10/1 -> Subsystem10/1
  Subsystem10/1 -> Add10/2, Product2/11
  Divide11/1 -> Interpreted MATLAB Function10/1
  Constant11/1 -> Add11/1
  Add11/1 -> Divide12/2
  Interpreted MATLAB Function11/1 -> Subsystem11/1
  Subsystem11/1 -> Add11/2, Product2/12
  Divide12/1 -> Interpreted MATLAB Function11/1
  Constant12/1 -> Add12/1
  Add12/1 -> Divide13/2
  Interpreted MATLAB Function12/1 -> Subsystem12/1
  Subsystem12/1 -> Add12/2, Product2/13
  Divide13/1 -> Interpreted MATLAB Function12/1
  Constant8/1 -> Add8/1
  Add8/1 -> Divide9/2
  Interpreted MATLAB Function8/1 -> Subsystem8/1
  Subsystem8/1 -> Add8/2, Product2/9
  Divide9/1 -> Interpreted MATLAB Function8/1
  Constant4/1 -> Add4/1
  Add4/1 -> Divide5/2
  Interpreted MATLAB Function4/1 -> Subsystem4/1
  Subsystem4/1 -> Add4/2, Product2/5
  Divide5/1 -> Interpreted MATLAB Function4/1
  Constant5/1 -> Add5/1
  Add5/1 -> Divide6/2
  Interpreted MATLAB Function5/1 -> Subsystem5/1
  Subsystem5/1 -> Add5/2, Product2/6
  Divide6/1 -> Interpreted MATLAB Function5/1
  Constant6/1 -> Add6/1
  Add6/1 -> Divide7/2
  Interpreted MATLAB Function6/1 -> Subsystem6/1
  Subsystem6/1 -> Add6/2, Product2/7
  Divide7/1 -> Interpreted MATLAB Function6/1
  Constant7/1 -> Add7/1
  Add7/1 -> Divide8/2
  Interpreted MATLAB Function7/1 -> Subsystem7/1
  Subsystem7/1 -> Add7/2, Product2/8
  Divide8/1 -> Interpreted MATLAB Function7/1
  Constant/1 -> Add/1
  Add/1 -> Divide1/2
  Interpreted MATLAB Function/1 -> Subsystem/1(In1)
  Subsystem/1(Out1) -> Add/2, Product2/1
  Divide1/1 -> Interpreted MATLAB Function/1
  Constant1/1 -> Add1/1
  Add1/1 -> Divide2/2
  Interpreted MATLAB Function1/1 -> Subsystem1/1
  Subsystem1/1 -> Add1/2, Product2/2
  Divide2/1 -> Interpreted MATLAB Function1/1
  Constant2/1 -> Add2/1
  Add2/1 -> Divide3/2
  Interpreted MATLAB Function2/1 -> Subsystem2/1
  Subsystem2/1 -> Product2/3, Add2/2
  Divide3/1 -> Interpreted MATLAB Function2/1
  Constant3/1 -> Add3/1
  Add3/1 -> Divide4/2
  Interpreted MATLAB Function3/1 -> Subsystem3/1
  Subsystem3/1 -> Product2/4, Add3/2
  Divide4/1 -> Interpreted MATLAB Function3/1
  Product2/1 -> Divide19/1, Divide20/1, Divide21/1, Divide22/1, Divide23/1, Divide24/1, Divide25/1, Divide34/1, Divide33/1, Divide32/1, Divide31/1, Divide29/1, Divide28/1, Divide27/1, Divide18/1, Divide30/1, Divide6/1, Divide7/1, Divide8/1, Divide9/1, Divide4/1, Divide3/1, Divide2/1, Divide1/1, Divide5/1, Divide10/1, Divide11/1, Divide12/1, Divide13/1, Divide14/1, Divide15/1, Divide16/1, Divide17/1
  Constant22/1 -> Add22/1
  Add22/1 -> Divide23/2
  Interpreted MATLAB Function22/1 -> Subsystem22/1
  Subsystem22/1 -> Product2/31, Add22/2
  Divide23/1 -> Interpreted MATLAB Function22/1
  Constant23/1 -> Add23/1
  Add23/1 -> Divide24/2
  Interpreted MATLAB Function23/1 -> Subsystem23/1
  Subsystem23/1 -> Product2/32, Add23/2
  Divide24/1 -> Interpreted MATLAB Function23/1
  Constant24/1 -> Add24/1
  Add24/1 -> Divide25/2
  Interpreted MATLAB Function24/1 -> Subsystem24/1
  Subsystem24/1 -> Product2/33, Add24/2
  Divide25/1 -> Interpreted MATLAB Function24/1
  Constant33/1 -> Add33/1
  Add33/1 -> Divide19/2
  Interpreted MATLAB Function33/1 -> Subsystem33/1
  Subsystem33/1 -> Product2/27, Add33/2
  Divide19/1 -> Interpreted MATLAB Function33/1
  Constant19/1 -> Add19/1
  Add19/1 -> Divide20/2
  Interpreted MATLAB Function19/1 -> Subsystem19/1
  Subsystem19/1 -> Product2/28, Add19/2
  Divide20/1 -> Interpreted MATLAB Function19/1
  Constant20/1 -> Add20/1
  Add20/1 -> Divide21/2
  Interpreted MATLAB Function20/1 -> Subsystem20/1
  Subsystem20/1 -> Product2/29, Add20/2
  Divide21/1 -> Interpreted MATLAB Function20/1
  Constant21/1 -> Add21/1
  Add21/1 -> Divide22/2
  Interpreted MATLAB Function21/1 -> Subsystem21/1
  Subsystem21/1 -> Product2/30, Add21/2
  Divide22/1 -> Interpreted MATLAB Function21/1
  Constant32/1 -> Add32/1
  Add32/1 -> Divide34/2
  Interpreted MATLAB Function32/1 -> Subsystem32/1
  Subsystem32/1 -> Product2/26, Add32/2
  Divide34/1 -> Interpreted MATLAB Function32/1
  Constant28/1 -> Add28/1
  Add28/1 -> Divide30/2
  Interpreted MATLAB Function28/1 -> Subsystem28/1
  Subsystem28/1 -> Product2/22, Add28/2
  Divide30/1 -> Interpreted MATLAB Function28/1
  Constant29/1 -> Add29/1
  Add29/1 -> Divide31/2
  Interpreted MATLAB Function29/1 -> Subsystem29/1
  Subsystem29/1 -> Product2/23, Add29/2
  Divide31/1 -> Interpreted MATLAB Function29/1
  Constant30/1 -> Add30/1
  Add30/1 -> Divide32/2
  Interpreted MATLAB Function30/1 -> Subsystem30/1
  Subsystem30/1 -> Product2/24, Add30/2
  Divide32/1 -> Interpreted MATLAB Function30/1
  Constant31/1 -> Add31/1
  Add31/1 -> Divide33/2
  Interpreted MATLAB Function31/1 -> Subsystem31/1
  Subsystem31/1 -> Product2/25, Add31/2
  Divide33/1 -> Interpreted MATLAB Function31/1
  Constant17/1 -> Add17/1
  Add17/1 -> Divide18/2
  Interpreted MATLAB Function17/1 -> Subsystem17/1
  Subsystem17/1 -> Product2/18, Add17/2
  Divide18/1 -> Interpreted MATLAB Function17/1
  Constant18/1 -> Add18/1
  Add18/1 -> Divide27/2
  Interpreted MATLAB Function18/1 -> Subsystem18/1
  Subsystem18/1 -> Product2/19, Add18/2
  Divide27/1 -> Interpreted MATLAB Function18/1
  Constant26/1 -> Add26/1
  Add26/1 -> Divide28/2
  Interpreted MATLAB Function26/1 -> Subsystem26/1
  Subsystem26/1 -> Product2/20, Add26/2
  Divide28/1 -> Interpreted MATLAB Function26/1
  Constant27/1 -> Add27/1
  Add27/1 -> Divide29/2
  Interpreted MATLAB Function27/1 -> Subsystem27/1
  Subsystem27/1 -> Product2/21, Add27/2
  Divide29/1 -> Interpreted MATLAB Function27/1
  connections:
  f_b_up13/RConn1 -- Subsystem12/RConn1
  f_b_up15/RConn1 -- Subsystem14/RConn1
  f_b_up16/RConn1 -- Subsystem15/RConn1
  f_b_up12/RConn1 -- Subsystem11/RConn1
  f_b_up17/RConn1 -- Subsystem16/RConn1
  f_b_up14/RConn1 -- Subsystem13/RConn1
  f_b_up11/RConn1 -- Subsystem10/RConn1
  f_b_up10/RConn1 -- Subsystem9/RConn1
  f_b_up9/RConn1 -- Subsystem8/RConn1
  f_b_up7/RConn1 -- Subsystem6/RConn1
  f_b_up8/RConn1 -- Subsystem7/RConn1
  f_b_up6/RConn1 -- Subsystem5/RConn1
  f_b_up5/RConn1 -- Subsystem4/RConn1
  f_b_up2/RConn1 -- Subsystem/RConn1
  f_b_up1/RConn1 -- Subsystem1/RConn1
  f_b_up3/RConn1 -- Subsystem2/RConn1
  f_b_up4/RConn1 -- Subsystem3/RConn1
  f_b_up31/RConn1 -- Subsystem22/RConn1
  f_b_up28/RConn1 -- Subsystem19/RConn1
  f_b_up21/RConn1 -- Subsystem27/RConn1
  f_b_up20/RConn1 -- Subsystem26/RConn1
  f_b_up30/RConn1 -- Subsystem21/RConn1
  f_b_up32/RConn1 -- Subsystem23/RConn1
  f_b_up33/RConn1 -- Subsystem24/RConn1
  f_b_up29/RConn1 -- Subsystem20/RConn1
  f_b_up27/RConn1 -- Subsystem33/RConn1
  f_b_up26/RConn1 -- Subsystem32/RConn1
  f_b_up24/RConn1 -- Subsystem30/RConn1
  f_b_up25/RConn1 -- Subsystem31/RConn1
  f_b_up23/RConn1 -- Subsystem29/RConn1
  f_b_up22/RConn1 -- Subsystem28/RConn1
  f_b_up18/RConn1 -- Subsystem17/RConn1
  f_b_up19/RConn1 -- Subsystem18/RConn1

== system LibFactorGraph/Diverter7 ==
  Add{,1..3} (4 alike) : Sum
  Constant{,1..3} (4 alike) : Constant  Value=epsVal
  Divide{1..4} (4 alike) : Product  Inputs=*/
  Interpreted MATLAB Function{,1..3} (4 alike) : MATLABFcn  MATLABFcn=fcn(u)  Output1D=off
  Product2 : Product  Inputs=4  RndMeth=Zero
  Subsystem : Subsystem
  Subsystem1 : LibFactorGraph/Diverter3/Subsystem
  Subsystem2 : LibFactorGraph/Diverter3/Subsystem
  Subsystem3 : LibFactorGraph/Diverter3/Subsystem
  f_b_up2 : PMIOPort  Port=1  Side=Left
  f_b_up1 : PMIOPort  Port=2  Side=Right
  f_b_up3 : PMIOPort  Port=3  Side=Left
  f_b_up4 : PMIOPort  Port=4  Side=Right
  wires:
  Constant/1 -> Add/1
  Add/1 -> Divide1/2
  Interpreted MATLAB Function/1 -> Subsystem/1(In1)
  Subsystem/1(Out1) -> Add/2, Product2/1
  Divide1/1 -> Interpreted MATLAB Function/1
  Constant1/1 -> Add1/1
  Add1/1 -> Divide2/2
  Interpreted MATLAB Function1/1 -> Subsystem1/1
  Subsystem1/1 -> Product2/2, Add1/2
  Divide2/1 -> Interpreted MATLAB Function1/1
  Constant2/1 -> Add2/1
  Add2/1 -> Divide3/2
  Interpreted MATLAB Function2/1 -> Subsystem2/1
  Subsystem2/1 -> Product2/3, Add2/2
  Divide3/1 -> Interpreted MATLAB Function2/1
  Constant3/1 -> Add3/1
  Add3/1 -> Divide4/2
  Interpreted MATLAB Function3/1 -> Subsystem3/1
  Subsystem3/1 -> Product2/4, Add3/2
  Divide4/1 -> Interpreted MATLAB Function3/1
  Product2/1 -> Divide4/1, Divide3/1, Divide2/1, Divide1/1
  connections:
  f_b_up2/RConn1 -- Subsystem/RConn1
  f_b_up1/RConn1 -- Subsystem1/RConn1
  f_b_up3/RConn1 -- Subsystem2/RConn1
  f_b_up4/RConn1 -- Subsystem3/RConn1

== system LibFactorGraph/Diverter8 ==
  Add : Sum
  Add1 : Sum
  Add2 : Sum
  Constant : Constant  Value=epsVal
  Constant1 : Constant  Value=epsVal
  Constant2 : Constant  Value=epsVal
  Divide1 : Product  Inputs=*/
  Divide2 : Product  Inputs=*/
  Divide3 : Product  Inputs=*/
  Interpreted MATLAB Function : MATLABFcn  MATLABFcn=fcn(u)  Output1D=off
  Interpreted MATLAB Function1 : MATLABFcn  MATLABFcn=fcn(u)  Output1D=off
  Interpreted MATLAB Function2 : MATLABFcn  MATLABFcn=fcn(u)  Output1D=off
  Product2 : Product  Inputs=3  RndMeth=Zero
  Subsystem : Subsystem
  Subsystem1 : LibFactorGraph/Diverter3/Subsystem
  Subsystem2 : LibFactorGraph/Diverter3/Subsystem
  f_b_up2 : PMIOPort  Port=1  Side=Left
  f_b_up1 : PMIOPort  Port=2  Side=Right
  f_b_up3 : PMIOPort  Port=3  Side=Left
  wires:
  Product2/1 -> Divide3/1, Divide1/1, Divide2/1
  Divide3/1 -> Interpreted MATLAB Function2/1
  Subsystem2/1 -> Add2/2, Product2/3
  Interpreted MATLAB Function2/1 -> Subsystem2/1
  Add2/1 -> Divide3/2
  Constant2/1 -> Add2/1
  Divide2/1 -> Interpreted MATLAB Function1/1
  Subsystem1/1 -> Add1/2, Product2/2
  Interpreted MATLAB Function1/1 -> Subsystem1/1
  Add1/1 -> Divide2/2
  Constant1/1 -> Add1/1
  Divide1/1 -> Interpreted MATLAB Function/1
  Subsystem/1(Out1) -> Product2/1, Add/2
  Interpreted MATLAB Function/1 -> Subsystem/1(In1)
  Add/1 -> Divide1/2
  Constant/1 -> Add/1
  connections:
  f_b_up3/RConn1 -- Subsystem2/RConn1
  f_b_up1/RConn1 -- Subsystem1/RConn1
  f_b_up2/RConn1 -- Subsystem/RConn1
